simulink model "current_model"  (R2025b)
settings: Solver=VariableStepAuto  StartTime=0.0  StopTime=10.0  RelTol=1e-3
undefined symbols (not defined in the file): L, R
settings Model: Creator=karadeli  LastModifiedBy=karadeli

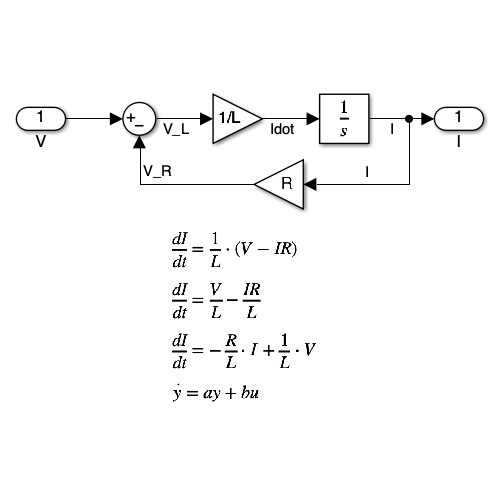
[thumbnail: Simulink's stored preview of the top-level diagram]
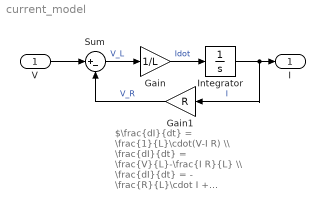
== system current_model ==
  note: $\frac{dI}{dt} = \frac{1}{L}\cdot(V-I R) \\ \frac{dI}{dt} = \frac{V}{L}-\frac{I R}{L} \\ \frac{dI}{dt} = - \frac{R}{L}\cdot I + \frac{1}{L}\cdot V \\ \dot{y}=ay+bu$
  V : Inport
  Gain : Gain  Gain=1/L
  Gain1 : Gain  Gain=R
  Integrator : Integrator
  Sum : Sum  Inputs=|+-
  I : Outport
  wires:
  V/1 -> Sum/1
  Sum/1 -> Gain/1  "V_L"
  Gain/1 -> Integrator/1  "Idot"
  Integrator/1 -> I/1, Gain1/1  "I"
  Gain1/1 -> Sum/2  "V_R"
